simulink model "relative_dynamics"  (R2021a)
settings: Solver=VariableStepAuto  StartTime=0.0  StopTime=time_sim  FixedStep=1  RelTol=1e-7  AbsTol=1e-9
undefined symbols (not defined in the file or in its folder): e, init_conds, init_conds_z, n, reference_conds
libraries: pid_lib x2
settings Model: Creator=danie  LastModifiedBy=danie
settings SolverCC: AlgebraicLoopSolver=TrustRegion
settings DebuggingCC: SFMachineParentedDataDiag=warning

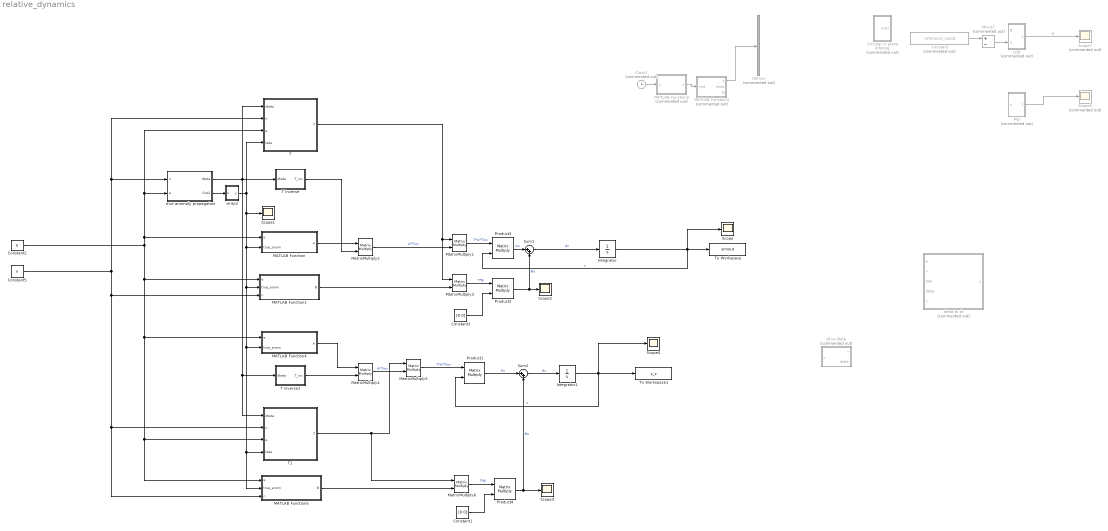
== system relative_dynamics ==
  Circular in plane orbiting : Subsystem  Commented=on
  Clock1 : Clock  Commented=on
  Constant : Constant  Commented=on  Value=reference_conds
  Constant1 : Constant  Value=[0 0]
  Constant2 : Constant  Value=e
  Constant3 : Constant  Value=[0 0]
  Constant5 : Constant  Value=n
  Demux : Demux  Commented=on  Outputs=6
  Integrator : Integrator  InitialCondition=init_conds
  Integrator1 : Integrator  InitialCondition=init_conds_z
  LQR : Subsystem  Commented=on
  MATLAB Function : MATLAB Function  TreatAsAtomicUnit=on
  MATLAB Function1 : MATLAB Function  TreatAsAtomicUnit=on
  MATLAB Function2 : MATLAB Function  Commented=on  TreatAsAtomicUnit=on
  MATLAB Function3 : MATLAB Function  Commented=on  TreatAsAtomicUnit=on
  MATLAB Function4 : MATLAB Function  TreatAsAtomicUnit=on
  MATLAB Function5 : MATLAB Function  TreatAsAtomicUnit=on
  MatrixMultiply{1..6} (6 alike) : Product  Multiplication=Matrix(*)
  Minus1 : Sum  Commented=on  Inputs=+-
  PID : Subsystem  Commented=on
  Product{1..4} (4 alike) : Product  SCDEnableBlockLinearizationSpecification=on  Multiplication=Matrix(*)
  Scope{,1..4} (5 alike) : Scope
  Scope5 : Scope  Commented=on
  Scope7 : Scope  Commented=on
  Sum1 : Sum  Inputs=|++
  Sum2 : Sum  Inputs=|++
  T : MATLAB Function  TreatAsAtomicUnit=on
  T inverse : MATLAB Function  TreatAsAtomicUnit=on
  T inverse1 : MATLAB Function  TreatAsAtomicUnit=on
  T1 : MATLAB Function  TreatAsAtomicUnit=on
  To Workspace : ToWorkspace  VariableName=simout  SaveFormat=Timeseries  SampleTime=-1
  To Workspace1 : ToWorkspace  VariableName=z_z  SaveFormat=Timeseries  SampleTime=-1
  dt to dteta : MATLAB Function  Commented=on  TreatAsAtomicUnit=on
  dteta to dt : MATLAB Function  Commented=on  TreatAsAtomicUnit=on
  true anomaly propagation : Subsystem
  wrap2 : MATLAB Function  TreatAsAtomicUnit=on
  wires:
  Constant5/1 -> MATLAB Function5/3(n), T1/2(n), MATLAB Function1/3(n), T/2(n), true anomaly propagation/1(n)
  MATLAB Function2/1(y) -> MATLAB Function3/1(mjd)
  MATLAB Function3/1(y) -> Demux/1
  Clock1/1 -> MATLAB Function2/1(u)
  Integrator/1 -> Scope/1, To Workspace/1, Product3/2  "x"
  Constant2/1 -> MATLAB Function5/1(e), T1/3(e), MATLAB Function4/1(e), MATLAB Function1/1(e), T/3(e), true anomaly propagation/2(e), MATLAB Function/1(e)
  LQR/1(Out1) -> Scope7/1  "u"
  Minus1/1 -> LQR/2(In2)
  Product3/1 -> Sum1/1  "Ax"
  Product2/1 -> Sum1/2, Scope2/1  "Bu"
  Constant/1 -> Minus1/1
  PID/1(Out1) -> Scope5/1
  Sum1/1 -> Integrator/1  "dx"
  Constant3/1 -> Product2/2
  true anomaly propagation/1(dteta) -> T inverse/1(dteta), T/1(dteta), T1/1(dteta), T inverse1/1(dteta)
  true anomaly propagation/2(Out2) -> wrap2/1(u)
  T/1(T) -> MatrixMultiply3/1, MatrixMultiply1/1
  MatrixMultiply1/1 -> Product3/1  "T*A*Tinv"
  T inverse/1(T_inv) -> MatrixMultiply2/2
  MATLAB Function1/1(B) -> MatrixMultiply3/2
  MATLAB Function/1(A) -> MatrixMultiply2/1
  MatrixMultiply2/1 -> MatrixMultiply1/2  "A*Tinv"
  wrap2/1(y) -> Scope1/1, MATLAB Function5/2(true_anom), T1/4(teta), MATLAB Function4/2(true_anom), MATLAB Function1/2(true_anom), MATLAB Function/2(true_anom), T/4(teta)
  MatrixMultiply3/1 -> Product2/1  "T*B"
  T inverse1/1(T_inv) -> MatrixMultiply4/2
  MATLAB Function4/1(A) -> MatrixMultiply4/1
  MatrixMultiply4/1 -> MatrixMultiply5/2  "A*Tinv"
  T1/1(T) -> MatrixMultiply6/1, MatrixMultiply5/1
  MatrixMultiply5/1 -> Product1/1  "T*A*Tinv"
  Product1/1 -> Sum2/1  "Ax"
  Sum2/1 -> Integrator1/1  "dx"
  Integrator1/1 -> Scope4/1, To Workspace1/1, Product1/2  "x"
  Product4/1 -> Scope3/1, Sum2/2  "Bu"
  Constant1/1 -> Product4/2
  MATLAB Function5/1(B) -> MatrixMultiply6/2
  MatrixMultiply6/1 -> Product4/1  "T*B"

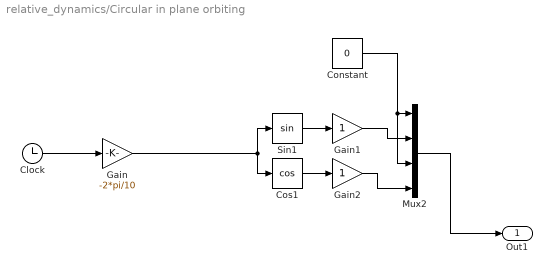
== system relative_dynamics/Circular in plane orbiting ==
  Clock : Clock
  Constant : Constant  Value=0
  Cos1 : Trigonometry  Operator=cos
  Gain : Gain  Gain=-2*pi/10
  Gain1 : Gain
  Gain2 : Gain
  Mux2 : Mux
  Sin1 : Trigonometry
  Out1 : Outport
  wires:
  Gain/1 -> Cos1/1, Sin1/1
  Gain2/1 -> Mux2/4
  Clock/1 -> Gain/1
  Sin1/1 -> Gain1/1
  Cos1/1 -> Gain2/1
  Mux2/1 -> Out1/1
  Gain1/1 -> Mux2/2
  Constant/1 -> Mux2/3, Mux2/1

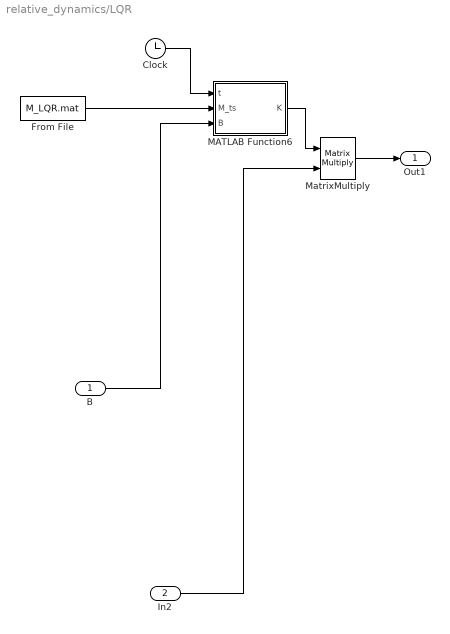
== system relative_dynamics/LQR ==
  B : Inport
  In2 : Inport  Port=2
  Clock : Clock
  From File : FromFile  FileName=M_LQR.mat  SampleTime=0
  MATLAB Function6 : MATLAB Function  TreatAsAtomicUnit=on
  MatrixMultiply : Product  Multiplication=Matrix(*)
  Out1 : Outport
  wires:
  MATLAB Function6/1(K) -> MatrixMultiply/1
  From File/1 -> MATLAB Function6/2(M_ts)
  Clock/1 -> MATLAB Function6/1(t)
  MatrixMultiply/1 -> Out1/1
  B/1 -> MATLAB Function6/3(B)
  In2/1 -> MatrixMultiply/2

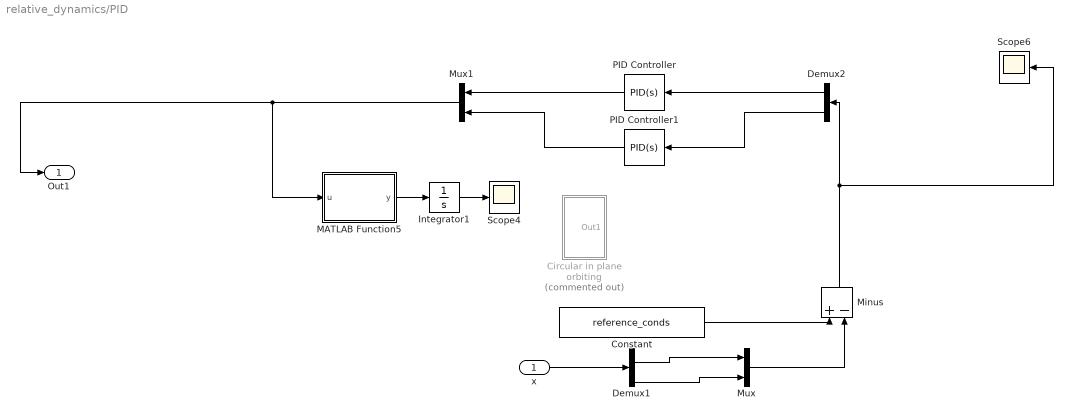
== system relative_dynamics/PID ==
  x : Inport
  Circular in plane orbiting : Subsystem  Commented=on
  Constant : Constant  Value=reference_conds
  Demux1 : Demux
  Demux2 : Demux  Outputs=2
  Integrator1 : Integrator
  MATLAB Function5 : MATLAB Function  TreatAsAtomicUnit=on
  Minus : Sum  Inputs=+-
  Mux : Mux  Inputs=2
  Mux1 : Mux  Inputs=2
  PID Controller : pid_lib/PID Controller  Controller=PID  Form=Parallel  TimeDomain=Continuous-time  UseExternalTs=off  SampleTime=-1  IntegratorMethod=Forward Euler  FilterMethod=Forward Euler  ControllerParametersSource=internal  P=124.255816056624  I=62.7356847110583  D=56.0069270493087  UseFilter=on  N=597.64677391099  TunerSelectOption=Transfer Function Based (PID Tuner App)  InitialConditionSource=internal  InitialConditionForIntegrator=0  InitialConditionForFilter=0  DifferentiatorICPrevScaledInput=0  ExternalReset=none  TrackingMode=off  Kt=1  LimitOutput=off  SatLimitsSource=internal  UpperSaturationLimit=inf  LowerSaturationLimit=-inf  LinearizeAsGain=on  AntiWindupMode=none  Kb=1  POutMin=[]  POutMax=[]  IOutMin=[]  IOutMax=[]  DOutMin=[]  DOutMax=[]  NOutMin=[]  NOutMax=[]  SumOutMin=[]  SumOutMax=[]  SaturationOutMin=[]  SaturationOutMax=[]  PParamMin=[]  PParamMax=[]  IParamMin=[]  IParamMax=[]  DParamMin=[]  DParamMax=[]  NParamMin=[]  NParamMax=[]  KbParamMin=[]  KbParamMax=[]  KtParamMin=[]  KtParamMax=[]  KbOutMin=[]  KbOutMax=[]  KtOutMin=[]  KtOutMax=[]  IntegratorOutMin=[]  IntegratorOutMax=[]  FilterOutMin=[]  FilterOutMax=[]  SumI1OutMin=[]  SumI1OutMax=[]  SumI2OutMin=[]  SumI2OutMax=[]  SumI3OutMin=[]  SumI3OutMax=[]  SumI4OutMin=[]  SumI4OutMax=[]  SumDOutMin=[]  SumDOutMax=[]  DifferentiatorOutMin=[]  DifferentiatorOutMax=[]  FilterDiffOutCoefMin=[]  FilterDiffOutCoefMax=[]  ReciprocalOutMin=[]  ReciprocalOutMax=[]  SumDenOutMin=[]  SumDenOutMax=[]  SumNumOutMin=[]  SumNumOutMax=[]  DivideOutMin=[]  DivideOutMax=[]  UdiffTsProdOutMin=[]  UdiffTsProdOutMax=[]  NTsProdOutMin=[]  NTsProdOutMax=[]  UintegralTsProdOutMin=[]  UintegralTsProdOutMax=[]  UngainTsProdOutMin=[]  UngainTsProdOutMax=[]  IntegratorContinuousStateAttributes=''  IntegratorStateMustResolveToSignalObject=off  IntegratorRTWStateStorageClass=Auto  FilterContinuousStateAttributes=''  FilterStateMustResolveToSignalObject=off  FilterRTWStateStorageClass=Auto  ParallelPVariant=InternalParameters  IdealPVariant=Disabled  IVariant=InternalParameters  DVariant=InternalParameters  IntegratorVariant=Continuous  SatVariant=Disabled  AWVariant=Passthrough  PCopyVariant=Disabled  TRVariant=Disabled  FdbkBlocksVariant=Forward  IdealPFdbkVariant=Disabled  SatFdbkVariant=Disabled  DerivativeFilterVariant=ContFilter  NVariant=InternalParameters  NCopyVariant=Disabled  FilterICVariant=InternalICsFilter  IntegratorICVariant=InternalICs  ExternalResetVariant=Disabled  TRSumVariant=Passthrough  SumFdbkVariant=Disabled  SumVariant=Sum_PID  TsampFilterVariant=InternalTs  TsampNgainVariant=Passthrough  TsampIntegralVariant=Passthrough  ExternalSaturationOutDataTypeStr=Inherit: Same as second input
  PID Controller1 : pid_lib/PID Controller  Controller=PID  Form=Parallel  TimeDomain=Continuous-time  UseExternalTs=off  SampleTime=-1  IntegratorMethod=Forward Euler  FilterMethod=Forward Euler  ControllerParametersSource=internal  P=2.68945569490569e-12  I=8.33834469369932e-12  D=1.7579804177667e-13  UseFilter=on  N=308.158049029344  TunerSelectOption=Transfer Function Based (PID Tuner App)  InitialConditionSource=internal  InitialConditionForIntegrator=0  InitialConditionForFilter=0  DifferentiatorICPrevScaledInput=0  ExternalReset=none  TrackingMode=off  Kt=1  LimitOutput=off  SatLimitsSource=internal  UpperSaturationLimit=inf  LowerSaturationLimit=-inf  LinearizeAsGain=on  AntiWindupMode=none  Kb=1  POutMin=[]  POutMax=[]  IOutMin=[]  IOutMax=[]  DOutMin=[]  DOutMax=[]  NOutMin=[]  NOutMax=[]  SumOutMin=[]  SumOutMax=[]  SaturationOutMin=[]  SaturationOutMax=[]  PParamMin=[]  PParamMax=[]  IParamMin=[]  IParamMax=[]  DParamMin=[]  DParamMax=[]  NParamMin=[]  NParamMax=[]  KbParamMin=[]  KbParamMax=[]  KtParamMin=[]  KtParamMax=[]  KbOutMin=[]  KbOutMax=[]  KtOutMin=[]  KtOutMax=[]  IntegratorOutMin=[]  IntegratorOutMax=[]  FilterOutMin=[]  FilterOutMax=[]  SumI1OutMin=[]  SumI1OutMax=[]  SumI2OutMin=[]  SumI2OutMax=[]  SumI3OutMin=[]  SumI3OutMax=[]  SumI4OutMin=[]  SumI4OutMax=[]  SumDOutMin=[]  SumDOutMax=[]  DifferentiatorOutMin=[]  DifferentiatorOutMax=[]  FilterDiffOutCoefMin=[]  FilterDiffOutCoefMax=[]  ReciprocalOutMin=[]  ReciprocalOutMax=[]  SumDenOutMin=[]  SumDenOutMax=[]  SumNumOutMin=[]  SumNumOutMax=[]  DivideOutMin=[]  DivideOutMax=[]  UdiffTsProdOutMin=[]  UdiffTsProdOutMax=[]  NTsProdOutMin=[]  NTsProdOutMax=[]  UintegralTsProdOutMin=[]  UintegralTsProdOutMax=[]  UngainTsProdOutMin=[]  UngainTsProdOutMax=[]  IntegratorContinuousStateAttributes=''  IntegratorStateMustResolveToSignalObject=off  IntegratorRTWStateStorageClass=Auto  FilterContinuousStateAttributes=''  FilterStateMustResolveToSignalObject=off  FilterRTWStateStorageClass=Auto  ParallelPVariant=InternalParameters  IdealPVariant=Disabled  IVariant=InternalParameters  DVariant=InternalParameters  IntegratorVariant=Continuous  SatVariant=Disabled  AWVariant=Passthrough  PCopyVariant=Disabled  TRVariant=Disabled  FdbkBlocksVariant=Forward  IdealPFdbkVariant=Disabled  SatFdbkVariant=Disabled  DerivativeFilterVariant=ContFilter  NVariant=InternalParameters  NCopyVariant=Disabled  FilterICVariant=InternalICsFilter  IntegratorICVariant=InternalICs  ExternalResetVariant=Disabled  TRSumVariant=Passthrough  SumFdbkVariant=Disabled  SumVariant=Sum_PID  TsampFilterVariant=InternalTs  TsampNgainVariant=Passthrough  TsampIntegralVariant=Passthrough  ExternalSaturationOutDataTypeStr=Inherit: Same as second input
  Scope4 : Scope
  Scope6 : Scope
  Out1 : Outport
  wires:
  Demux2/1 -> PID Controller/1
  MATLAB Function5/1(y) -> Integrator1/1
  Mux1/1 -> Out1/1, MATLAB Function5/1(u)
  Mux/1 -> Minus/2
  Integrator1/1 -> Scope4/1
  Demux1/4 -> Mux/2
  Minus/1 -> Demux2/1, Scope6/1
  PID Controller/1 -> Mux1/1
  PID Controller1/1 -> Mux1/2
  Demux2/2 -> PID Controller1/1
  Demux1/2 -> Mux/1
  x/1 -> Demux1/1
  Constant/1 -> Minus/1

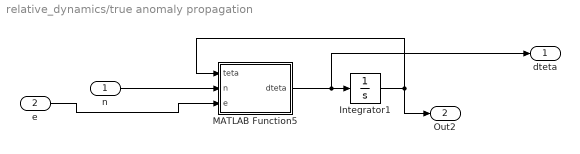
== system relative_dynamics/true anomaly propagation ==
  n : Inport
  e : Inport  Port=2
  Integrator1 : Integrator
  MATLAB Function5 : MATLAB Function  TreatAsAtomicUnit=on
  dteta : Outport
  Out2 : Outport  Port=2
  wires:
  MATLAB Function5/1(dteta) -> dteta/1, Integrator1/1
  e/1 -> MATLAB Function5/3(e)
  Integrator1/1 -> Out2/1, MATLAB Function5/1(teta)
  n/1 -> MATLAB Function5/2(n)

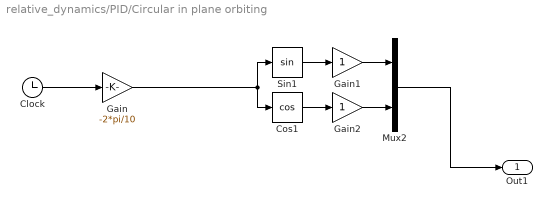
== system relative_dynamics/PID/Circular in plane orbiting ==
  Clock : Clock
  Cos1 : Trigonometry  Operator=cos
  Gain : Gain  Gain=-2*pi/10
  Gain1 : Gain
  Gain2 : Gain
  Mux2 : Mux  Inputs=2
  Sin1 : Trigonometry
  Out1 : Outport
  wires:
  Gain/1 -> Cos1/1, Sin1/1
  Gain2/1 -> Mux2/2
  Clock/1 -> Gain/1
  Sin1/1 -> Gain1/1
  Cos1/1 -> Gain2/1
  Mux2/1 -> Out1/1
  Gain1/1 -> Mux2/1

== matlab function relative_dynamics/T inverse ==
  data: dteta input; T_inv output
function T_inv = fcn(dteta)
T_inv=[1/dteta 0 0 0; 0 1 0 0; 0 0 1/dteta 0; 0 0 0 1];

== matlab function relative_dynamics/MATLAB Function1 ==
  data: e input; B output; true_anom input; n input
function B = B_ss(e,true_anom,n)
B=((1-(e^2))^3)/(((1+e*cos(true_anom))^4)*(n^2))*[1 0; 0 0; 0 1; 0 0];

== matlab function relative_dynamics/MATLAB Function4 ==
  data: e input; A output; true_anom input
function A = A_ss_z(e,true_anom)
A=[2*e*sin(true_anom)/(1+e*cos(true_anom)) -1/(1+e*cos(true_anom)); 1 0];

== matlab function relative_dynamics/T inverse1 ==
  data: dteta input; T_inv output
function T_inv = fcn(dteta)
T_inv=[1/dteta 0; 0 1;];

== matlab function relative_dynamics/T1 ==
  data: dteta input; T output; n input; e input; teta input
function T = fcn(dteta, n,e,teta)
T=[dteta^2 dteta*(-(n*2*(1+e*cos(teta))*e*sin(teta)/((1-e^2)^1.5))); 0 dteta];

== matlab function relative_dynamics/MATLAB Function5 ==
  data: e input; B output; true_anom input; n input
function B = B_ss(e,true_anom,n)
B=((1-(e^2))^3)/(((1+e*cos(true_anom))^4)*(n^2))*[1 0; 0 0];

== matlab function relative_dynamics/MATLAB Function ==
  data: e input; A output; true_anom input
function A = A_ss(e,true_anom)
A=[ 2*e*sin(true_anom)/(1+e*cos(true_anom)), (3+e*cos(true_anom))/(1+e*cos(true_anom)), 2, -2*e*sin(true_anom)/(1+e*cos(true_anom)); 
    1, 0, 0, 0;
   -2, 2*e*sin(true_anom)/(1+e*cos(true_anom)), 2*e*sin(true_anom)/(1+e*cos(true_anom)), e*cos(true_anom)/(1+e*cos(true_anom));
   0, 0, 1, 0];

== matlab function relative_dynamics/MATLAB Function2 ==
  data: u input; y output
function y = time_conv(u)
y=double(60676+((u/3600)/24));

== matlab function relative_dynamics/MATLAB Function3 ==
  data: mjd input; y output; mass output; M output
function [y, mass, M]= get_eph(mjd)
    [y, mass, M]=ephNEO(mjd,28);

== matlab function relative_dynamics/T ==
  data: dteta input; T output; n input; e input; teta input
function T = fcn(dteta, n,e,teta)
T=[dteta^2 dteta*(-(n*2*(1+e*cos(teta))*e*sin(teta)/((1-e^2)^1.5))) 0 0; 0 dteta 0 0; 0 0 dteta^2 dteta*(-(n*2*(1+e*cos(teta))*e*sin(teta)/((1-e^2)^1.5))); 0 0 0 dteta];

== matlab function relative_dynamics/PID/MATLAB Function5 ==
  data: u input; y output
function y = fcn(u)

y =norm(u);

== matlab function relative_dynamics/LQR/MATLAB Function6 ==
  data: t input; M_ts input; K output; B input
function K = fcn(t,M_ts,B)
flag=0;
% for i=1:(length(M_ts.Time)-1)
%     if and(t>=M_ts.Time(i),t<M_ts.Time(i+1))
%         M=M_ts.data(i);
%         flag=1;
%         break
%     else
%         M=zeros(4,4)
%     end
% end
M=reshape(M_ts,4,4);
K=-B.'*M;

== matlab function relative_dynamics/true anomaly propagation/MATLAB Function5 ==
  data: teta input; n input; dteta output; e input
function dteta = fcn(teta,n,e)
dteta=(n*(1+e*cos(teta))^2)/((1-e^2)^1.5);

== matlab function relative_dynamics/dteta to dt ==
  data: e input; y output; n input; teta input; dteta input; x input
function y = fcn(e,n,teta,dteta,x)
y=x;
y(1)=x(1)*(dteta^2)+dteta*(-(n*2*(1+e*cos(teta))*e*sin(teta)/((1-e^2)^1.5)))*x(2);
y(2)=x(2)*dteta;
y(3)=x(3)*(dteta^2)+dteta*(-(n*2*(1+e*cos(teta))*e*sin(teta)/((1-e^2)^1.5)))*x(4);
y(4)=x(4)*dteta;

== matlab function relative_dynamics/dt to dteta ==
  data: x input; y output; dteta input
function y = fcn(x,dteta)
y=x;
y(1)=x(1)/dteta;
y(3)=x(3)/dteta;

== matlab function relative_dynamics/wrap2 ==
  data: u input; y output
function y = fcn(u)

y = mod(u,2*pi);
